simulink model "state_space"  (R2018a)
settings: Solver=VariableStepAuto  StartTime=0.0  StopTime=10.0  RelTol=1e-3
settings Model: Creator=bssho  LastModifiedBy=bssho

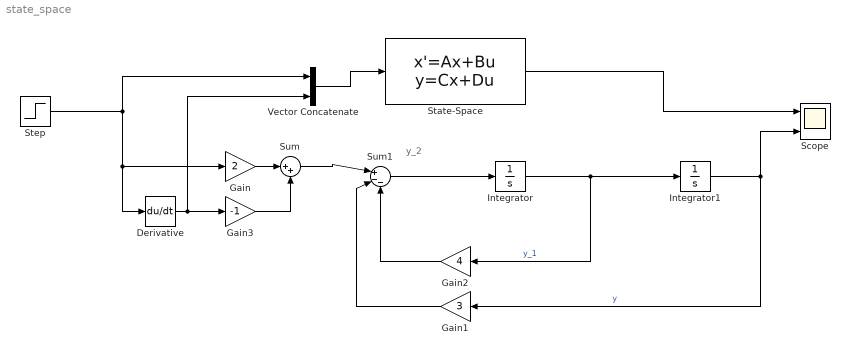
== system state_space ==
  note: y_2
  Derivative : Derivative
  Gain : Gain  Gain=2
  Gain1 : Gain  Gain=3
  Gain2 : Gain  Gain=4
  Gain3 : Gain  Gain=-1
  Integrator : Integrator  InitialCondition=1
  Integrator1 : Integrator
  Scope : Scope  NumInputPorts=2
  State-Space : StateSpace  A=[0 1 ; -3 -4]  B=[0 0 ; 2 -1]  C=[1 0]  D=[0 0]  InitialCondition=[0.5 0]
  Step : Step  Time=0  SampleTime=0
  Sum : Sum  Inputs=|++
  Sum1 : Sum  Inputs=|+--
  Vector Concatenate : Concatenate
  wires:
  Gain/1 -> Sum/1
  Integrator/1 -> Integrator1/1, Gain2/1  "y_1"
  Sum1/1 -> Integrator/1
  Integrator1/1 -> Scope/2, Gain1/1  "y"
  Sum/1 -> Sum1/1
  State-Space/1 -> Scope/1
  Vector Concatenate/1 -> State-Space/1
  Step/1 -> Gain/1, Derivative/1, Vector Concatenate/1
  Gain2/1 -> Sum1/3
  Gain1/1 -> Sum1/2
  Derivative/1 -> Gain3/1, Vector Concatenate/2
  Gain3/1 -> Sum/2
